simulink model "fig2_31_simulink"  (R2021b)
settings: Solver=ode45  StartTime=0.0  StopTime=9  RelTol=1e-3  EnableMultiTasking=on
settings Model: Creator=One Informatic  LastModifiedBy=One Informatic
settings DataIOCC: LimitDataPoints=on  SaveFormat=Array  SignalLoggingSaveFormat=ModelDataLogs  ReturnWorkspaceOutputs=off  SignalLoggingName=sigsOut
settings DebuggingCC: SaveWithParameterizedLinksMsg=none  UnderspecifiedInitializationDetection=Classic  MergeDetectMultiDrivingBlocksExec=none  SignalResolutionControl=TryResolveAllWithWarning  MultiTaskDSMMsg=warning  MultiTaskCondExecSysMsg=none
settings HardwareCC: ProdBitPerPointer=32  ProdBitPerSizeT=32  ProdBitPerPtrDiffT=32  ProdLargestAtomicFloat=None  ProdIntDivRoundTo=Undefined  ProdEndianess=Unspecified  ProdWordSize=32  ProdHWDeviceType=32-bit Generic  TargetUnknown=on
settings ModelReferenceCC: PropagateSignalLabelsOutOfModel=off
settings GRTTargetCC: CombineOutputUpdateFcns=off  GRTInterface=on
settings ConfigComp: CovMetricSettings=dw  CovSaveCumulativeToWorkspaceVar=on  CovSaveSingleToWorkspaceVar=on

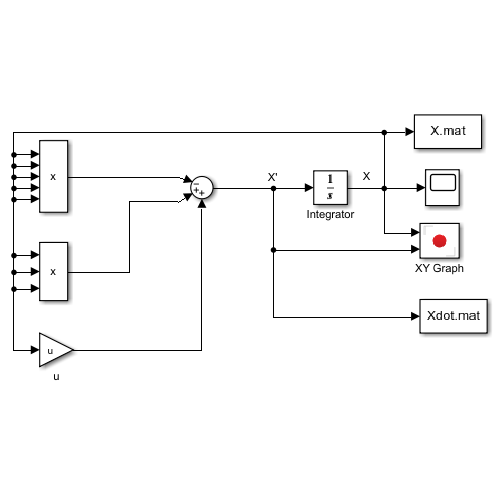
[thumbnail: Simulink's stored preview of the top-level diagram]
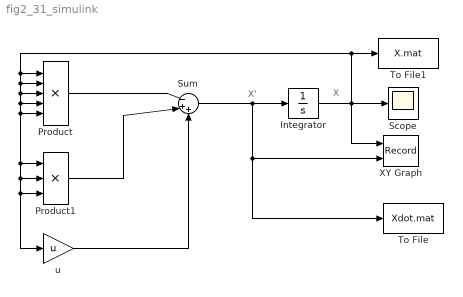
== system fig2_31_simulink ==
  note: X'
  note: X
  Integrator : Integrator  InitialCondition=-0.5
  Product : Product  Inputs=5
  Product1 : Product  Inputs=3
  Scope : Scope
  Sum : Sum  Inputs=|-++
  To File : ToFile  Filename=Xdot.mat  MatrixName=Xdot  SampleTime=0.001
  To File1 : ToFile  Filename=X.mat  MatrixName=X  SampleTime=0.001
  XY Graph : Record  FileSettingsInternal="{\"entries\":[{\"content\":{\"excelSettings\":{\"content\":{},\"type\":\"Streamout.ExcelSettings\"}},\"type\":\"Streamout.FileSettingStorage\",\"uuid\":\"6c3b332e-3c62-4d45-88eb-e11fe2c47eab\"}],\"packageUris\":[\"http://schema.mathworks.com/mf0/streamout_blocks/R2020a\"],\"version\":\"1.0\"}"  Layout=[1 1]  SignalsInternal="{\"entries\":[{\"content\":{\"signals\":[{\"content\":{\"blockPath\":[\"fig2_31_simulink/XY Graph\"],\"channel\":[],\"dimensions\":[1],\"domain\":\"fig2_31_simulink/XY Graph\",\"lineColor\":\"#a2142f\",\"plots\":[1],\"port\":1,\"sid\":[\"\"],\"signalID\":116336,\"signalName\":\"Integrator\"},\"type\":\"RecordBlkView.Signal\",\"uuid\":\"d667e41f-b18e-4329-98e1-6828f61dc8e3\"},{\"content\":{\"blockPath\":[\"fig2_31_simulink/XY Graph\"],\"channel\":[],\"dimensions\":[1],\"domain\":\"fig2_31_simulink/XY Graph\",\"lineColor\":\"#139fff\",\"plots\":[1],\"port\":2,\"sid\":[\"\"],\"signalID\":116340,\"signalName\":\"Sum\"},\"type\":\"RecordBlkView.Signal\",\"uuid\":\"b3a5fbec-d58c-4f69-b7e9-93409c420f6c\"}]},\"type\":\"RecordBlkView.InputSignals\",\"uuid\":\"8f253460-e8c5-4995-a5af-2a9c62523c61\"}],\"packageUris\":[\"http://schema.mathworks.com/mf0/streamout_blocks/R2020a\"],\"version\":\"1.0\"}"  VisualizationBindings="{\"xyplotplugin\":{\"info\":[{\"series\":[{\"bindingParametersList\":[{\"parameter\":\"X-Axis\",\"signalID\":116336,\"signalName\":\"Integrator\"},{\"parameter\":\"Y-Axis\",\"signalID\":116340,\"signalName\":\"Sum\"}],\"seriesID\":34164}],\"subplotID\":1}]}}"  CompatibilityTag=XY
  u : Gain  Gain=u
  wires:
  u/1 -> Sum/3
  Product1/1 -> Sum/2
  Product/1 -> Sum/1
  Sum/1 -> To File/1, XY Graph/2, Integrator/1
  Integrator/1 -> XY Graph/1, To File1/1, Product/1, u/1, Product1/3, Product1/2, Product1/1, Product/5, Product/4, Product/3, Product/2, Scope/1
